simulink model "ME471_Lab_Simulink"  (R2018b)
settings: Solver=FixedStepAuto  StartTime=0.0  StopTime=inf  FixedStep=0.001  RelTol=1e-3
values from neighbouring files (symbols this model uses):
  B = 0.001    [ME471_Lab.m]
  beta = double(beta)    [ME471_Lab.m]
  imax = 4.1    [ME471_Lab.m]
  K = imax*beta/(Ka*theta0)    [ME471_Lab.m]
  Ka = 0.41    [ME471_Lab.m]
  Km = 0.11    [ME471_Lab.m]
  Kp = 0.0458    [ME471_Lab.m]
  T = double(T)    [ME471_Lab.m]
  taum = J/B    (= 0.34)    [ME471_Lab.m]
libraries: sldrtlib x1
settings Model: Creator=Khrisna Adi Kamarga  LastModifiedBy=Khrisna Adi Kamarga

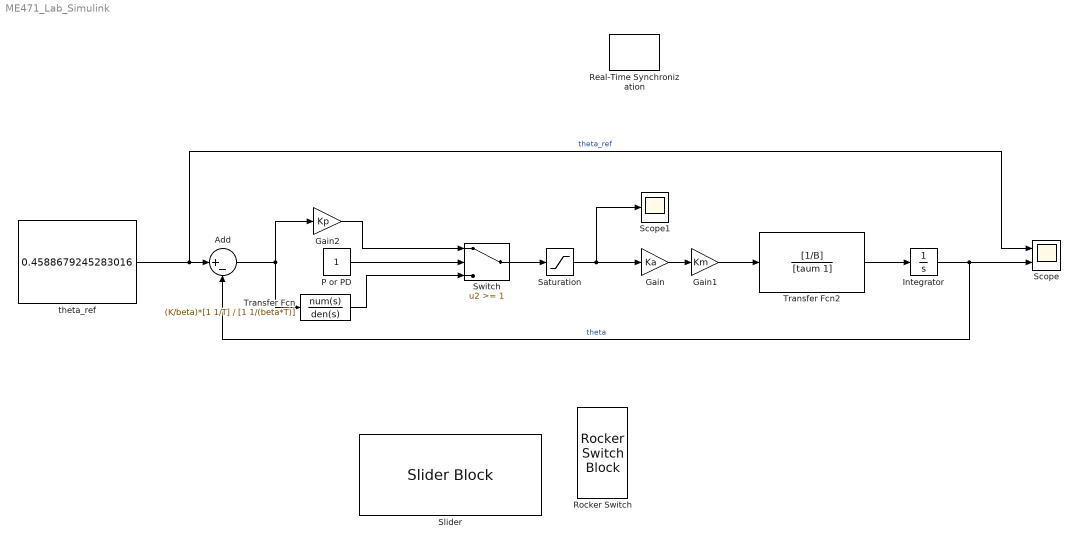
== system ME471_Lab_Simulink ==
  Add : Sum  Inputs=|+-
  Gain : Gain  Gain=Ka
  Gain1 : Gain  Gain=Km
  Gain2 : Gain  Gain=Kp
  Integrator : Integrator
  P or PD : Constant
  Real-Time Synchronization : sldrtlib/Real-Time Synchronization  SampleTime=0.01  MaxMissedTicks=100  ShowMissedTicks=off  YieldWhenWaiting=off
  Rocker Switch : RockerSwitchBlock  WebBlockId=18
      settings: Values={{'Off', 'On'}, [0 1]}
  Saturation : Saturate  UpperLimit=imax/Ka  LowerLimit=-imax/Ka
  Scope : Scope  NumInputPorts=2
  Scope1 : Scope
  Slider : SliderBlock  WebBlockId=12  ScaleMin=-3.2000000000000002  ScaleMax=3.2000000000000002
  Switch : Switch  Threshold=1
  Transfer Fcn : TransferFcn  Numerator=(K/beta)*[1 1/T]  Denominator=[1 1/(beta*T)]
  Transfer Fcn2 : TransferFcn  Numerator=[1/B]  Denominator=[taum 1]
  theta_ref : Constant  Value=0.4588679245283016
  wires:
  Gain/1 -> Gain1/1
  Transfer Fcn2/1 -> Integrator/1
  Integrator/1 -> Scope/2, Add/2  "theta"
  theta_ref/1 -> Scope/1, Add/1  "theta_ref"
  Transfer Fcn/1 -> Switch/3
  Add/1 -> Transfer Fcn/1, Gain2/1
  Gain2/1 -> Switch/1
  P or PD/1 -> Switch/2
  Gain1/1 -> Transfer Fcn2/1
  Switch/1 -> Saturation/1
  Saturation/1 -> Scope1/1, Gain/1
